simulink model "local_mins"  (R2018a)
settings: Solver=VariableStepDiscrete  StartTime=0.0  StopTime=100  RelTol=1e-3  EnableMultiTasking=on
settings Model: Creator=jrivitus  LastModifiedBy=bneiswan
settings DataIOCC: LimitDataPoints=on  SaveFormat=Array
settings OptimizationCC: ExpressionDepthLimit=2147483647  LifeSpan=inf
settings DebuggingCC: UnderspecifiedInitializationDetection=Classic  MergeDetectMultiDrivingBlocksExec=none  ParameterPrecisionLossMsg=none  AllowSymbolicDim=off  StateNameClashWarn=warning  SFUnexpectedBacktrackingDiag=warning  SFNoUnconditionalDefaultTransitionDiag=warning  SFExecutionAtInitializationDiag=none
settings HardwareCC: ProdBitPerPointer=32  ProdBitPerSizeT=32  ProdBitPerPtrDiffT=32  ProdLargestAtomicFloat=None  ProdIntDivRoundTo=Undefined  ProdEndianess=Unspecified  ProdWordSize=32  ProdHWDeviceType=32-bit Generic
settings ModelReferenceCC: PropagateSignalLabelsOutOfModel=off
settings CodeAppCC: StateflowObjectComments=on
settings GRTTargetCC: TargetLangStandard=C89/C90 (ANSI)  GeneratePreprocessorConditionals=Disable all
settings ConfigComp: CovMetricSettings=dw  CovHtmlReporting=on  CovSaveCumulativeToWorkspaceVar=on  CovSaveSingleToWorkspaceVar=on  CovExternalEMLEnable=off  CovSFcnEnable=off

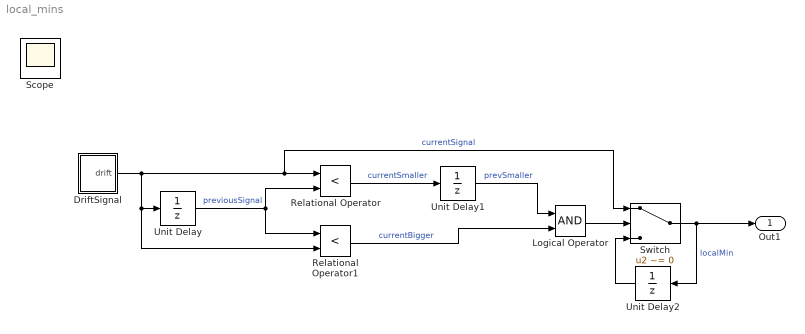
== system local_mins ==
  DriftSignal : Subsystem  TreatAsAtomicUnit=on  SystemSampleTime=1
  Logical Operator : Logic  AllPortsSameDT=off  OutDataTypeStr=boolean
  Relational Operator : RelationalOperator  Operator=<  OutDataTypeStr=boolean  RndMeth=Nearest
  Relational Operator1 : RelationalOperator  Operator=<  OutDataTypeStr=boolean  RndMeth=Nearest
  Switch : Switch  Criteria=u2 ~= 0
  Unit Delay : UnitDelay  SampleTime=-1
  Unit Delay1 : UnitDelay
  Unit Delay2 : UnitDelay
  Out1 : Outport
  Scope : Scope
  wires:
  Unit Delay1/1 -> Logical Operator/1  "prevSmaller"
  Relational Operator/1 -> Unit Delay1/1  "currentSmaller"
  Unit Delay/1 -> Relational Operator/2, Relational Operator1/1  "previousSignal"
  Relational Operator1/1 -> Logical Operator/2  "currentBigger"
  Logical Operator/1 -> Switch/2
  DriftSignal/1(drift) -> Relational Operator1/2, Unit Delay/1, Relational Operator/1, Switch/1  "currentSignal"
  Switch/1 -> Out1/1, Unit Delay2/1  "localMin"
  Unit Delay2/1 -> Switch/3

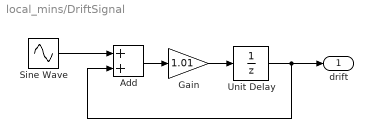
== system local_mins/DriftSignal ==
  Add : Sum
  Gain : Gain  Gain=1.01
  Sine Wave : Sin  Frequency=2*pi/10.3  SampleTime=1
  Unit Delay : UnitDelay
  drift : Outport
  wires:
  Unit Delay/1 -> drift/1, Add/2
  Sine Wave/1 -> Add/1
  Add/1 -> Gain/1
  Gain/1 -> Unit Delay/1
